simulink model "vel_pose_connect_sl"  (R2018b)
settings: Solver=VariableStepAuto  StartTime=0.0  StopTime=inf  RelTol=1e-3
undefined symbols (not defined in the file or in its folder): Angle, Brakepedal, Drivemode, Drivepedal, Gearshift, Header, Lamp, Light, Speed, Steeringmode, Tm, Twist
libraries: robotlib x19, simulink x3
settings Model: Creator=handai  LastModifiedBy=sdd

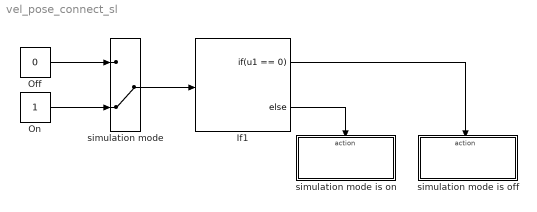
== system vel_pose_connect_sl ==
  If1 : If  IfExpression=u1 == 0
  Off : Constant  Value=0
  On : Constant
  simulation mode : ManualSwitch  CurrentSetting=0
  simulation mode is off : Subsystem  TreatAsAtomicUnit=on
  simulation mode is on : Subsystem  TreatAsAtomicUnit=on
  wires:
  Off/1 -> simulation mode/1
  On/1 -> simulation mode/2
  simulation mode/1 -> If1/1
  If1/1 -> simulation mode is off/Action
  If1/2 -> simulation mode is on/Action

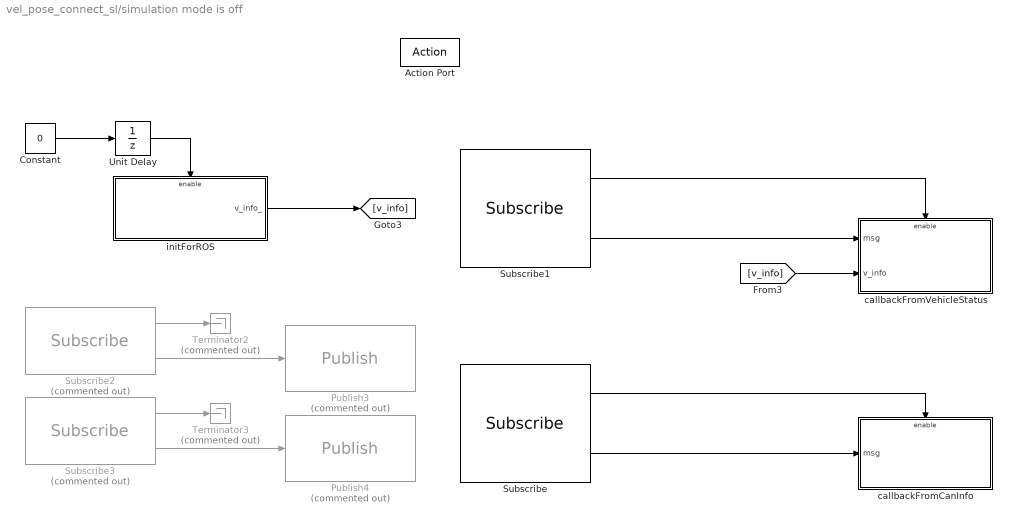
== system vel_pose_connect_sl/simulation mode is off ==
  Action Port : ActionPort  ActionType=then
  Constant : Constant  Value=0
  Publish3 : robotlib/Publish  Commented=on  topicSource=Specify your own  topic=/current_pose  messageType=geometry_msgs/PoseStamped  messageQueueLength=1
      settings: SourceProductBaseCode=RO
  Publish4 : robotlib/Publish  Commented=on  topicSource=Specify your own  topic=/current_velocity  messageType=geometry_msgs/TwistStamped  messageQueueLength=1
      settings: SourceProductBaseCode=RO
  Subscribe : robotlib/Subscribe  topicSource=Specify your own  topic=/can_info  messageType=autoware_msgs/CanInfo  sampleTime=-1  messageQueueLength=1
      settings: SourceProductBaseCode=RO
  Subscribe1 : robotlib/Subscribe  topicSource=Specify your own  topic=/vehicle_status  messageType=autoware_msgs/VehicleStatus  sampleTime=-1  messageQueueLength=1
      settings: SourceProductBaseCode=RO
  Subscribe2 : robotlib/Subscribe  Commented=on  topicSource=Specify your own  topic=/ndt_pose  messageType=geometry_msgs/PoseStamped  sampleTime=-1  messageQueueLength=1
      settings: SourceProductBaseCode=RO
  Subscribe3 : robotlib/Subscribe  Commented=on  topicSource=Specify your own  topic=/estimate_twist  messageType=geometry_msgs/TwistStamped  sampleTime=-1  messageQueueLength=1
      settings: SourceProductBaseCode=RO
  Terminator2 : Terminator  Commented=on
  Terminator3 : Terminator  Commented=on
  Unit Delay : UnitDelay  InitialCondition=1  SampleTime=-1
  callbackFromCanInfo : Subsystem
  callbackFromVehicleStatus : Subsystem
  initForROS : Subsystem
  wires:
  Subscribe2/2 -> Publish3/1
  Subscribe3/2 -> Publish4/1
  Subscribe2/1 -> Terminator2/1
  Subscribe3/1 -> Terminator3/1
  Subscribe/2 -> callbackFromCanInfo/1(msg)
  Subscribe/1 -> callbackFromCanInfo/Enable
  Subscribe1/2 -> callbackFromVehicleStatus/1(msg)
  Subscribe1/1 -> callbackFromVehicleStatus/Enable
  [v_info] -> callbackFromVehicleStatus/2(v_info)
  Constant/1 -> Unit Delay/1
  initForROS/1(v_info_) -> [v_info]
  Unit Delay/1 -> initForROS/Enable

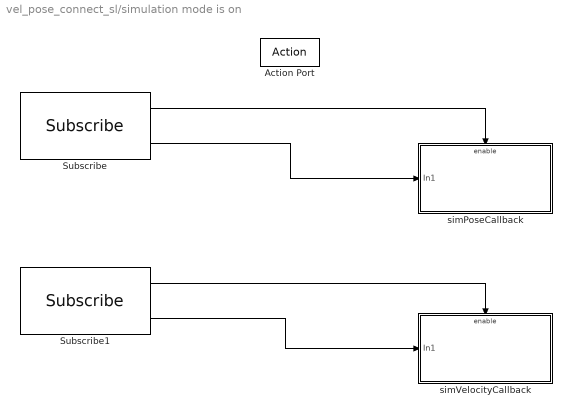
== system vel_pose_connect_sl/simulation mode is on ==
  Action Port : ActionPort  ActionType=else
  Subscribe : robotlib/Subscribe  topicSource=Specify your own  topic=/sim_pose  messageType=geometry_msgs/PoseStamped  sampleTime=-1  messageQueueLength=1
      settings: SourceProductBaseCode=RO
  Subscribe1 : robotlib/Subscribe  topicSource=Specify your own  topic=/sim_velocity  messageType=geometry_msgs/TwistStamped  sampleTime=-1  messageQueueLength=1
      settings: SourceProductBaseCode=RO
  simPoseCallback : Subsystem
  simVelocityCallback : Subsystem
  wires:
  Subscribe/1 -> simPoseCallback/Enable
  Subscribe1/1 -> simVelocityCallback/Enable
  Subscribe/2 -> simPoseCallback/1(In1)
  Subscribe1/2 -> simVelocityCallback/1(In1)

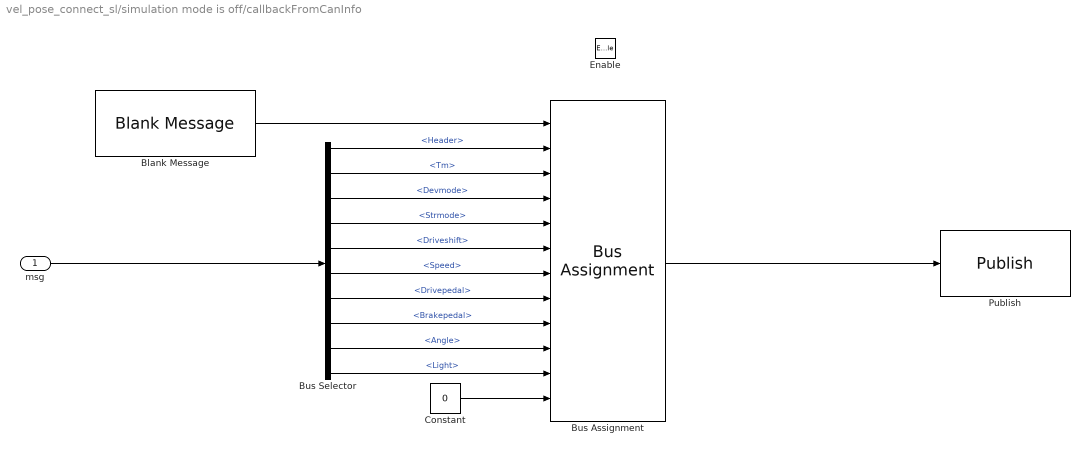
== system vel_pose_connect_sl/simulation mode is off/callbackFromCanInfo ==
  msg : Inport
  Enable : EnablePort
  Blank Message : robotlib/Blank Message  messageClass=Message  entityType=autoware_msgs/VehicleStatus  messageType=autoware_msgs/VehicleStatus  SampleTime=inf
      settings: SourceProductBaseCode=RO
  Bus Assignment : BusAssignment  AssignedSignals=Header,Tm,Drivemode,Steeringmode,Gearshift,Speed,Drivepedal,Brakepedal,Angle,Light,Lamp
  Bus Selector : BusSelector  OutputSignals=Header,Tm,Devmode,Strmode,Driveshift,Speed,Drivepedal,Brakepedal,Angle,Light
  Constant : Constant  Value=0  OutDataTypeStr=int32
  Publish : robotlib/Publish  topicSource=Specify your own  topic=/vehicle_status  messageType=autoware_msgs/VehicleStatus  messageQueueLength=1
      settings: SourceProductBaseCode=RO
  wires:
  Bus Selector/10 -> Bus Assignment/11  "<Light>"
  Bus Assignment/1 -> Publish/1
  Bus Selector/3 -> Bus Assignment/4  "<Devmode>"
  Bus Selector/5 -> Bus Assignment/6  "<Driveshift>"
  msg/1 -> Bus Selector/1
  Bus Selector/2 -> Bus Assignment/3  "<Tm>"
  Bus Selector/1 -> Bus Assignment/2  "<Header>"
  Constant/1 -> Bus Assignment/12
  Bus Selector/9 -> Bus Assignment/10  "<Angle>"
  Bus Selector/6 -> Bus Assignment/7  "<Speed>"
  Bus Selector/7 -> Bus Assignment/8  "<Drivepedal>"
  Bus Selector/8 -> Bus Assignment/9  "<Brakepedal>"
  Bus Selector/4 -> Bus Assignment/5  "<Strmode>"
  Blank Message/1 -> Bus Assignment/1

== system vel_pose_connect_sl/simulation mode is off/callbackFromVehicleStatus ==
  msg : Inport
  v_info : Inport  Port=2
  Enable : EnablePort
  publishVelocity : Subsystem  TreatAsAtomicUnit=on
  publishVelocityViz : Subsystem  TreatAsAtomicUnit=on
  wires:
  msg/1 -> publishVelocity/1(msg), publishVelocityViz/1(msg)
  v_info/1 -> publishVelocity/2(v_info)

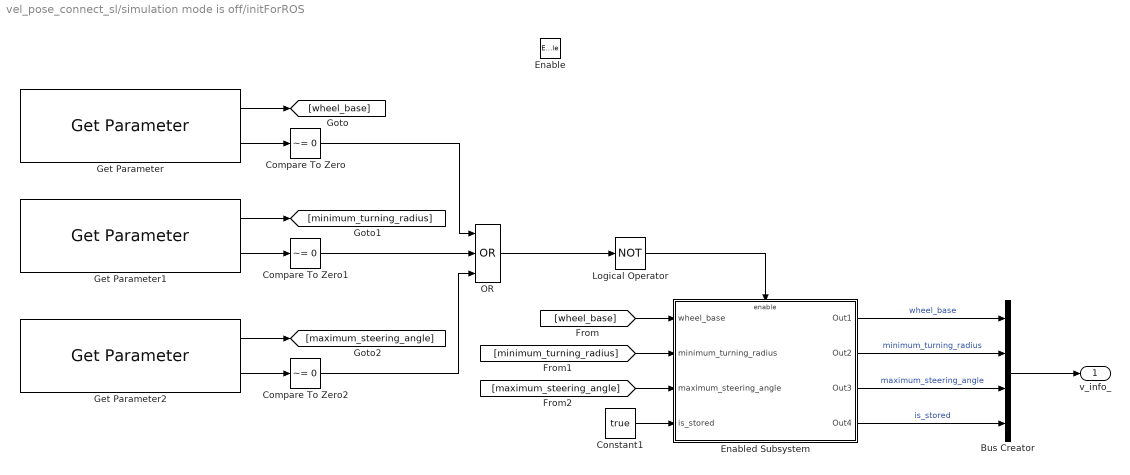
== system vel_pose_connect_sl/simulation mode is off/initForROS ==
  Enable : EnablePort
  Bus Creator : BusCreator  Inputs=4
  Compare To Zero : simulink/Logic and Bit Operations/Compare To Zero  relop=~=  OutDataTypeStr=boolean
  Compare To Zero1 : simulink/Logic and Bit Operations/Compare To Zero  relop=~=  OutDataTypeStr=boolean
  Compare To Zero2 : simulink/Logic and Bit Operations/Compare To Zero  relop=~=  OutDataTypeStr=boolean
  Constant1 : Constant  Value=true  OutDataTypeStr=boolean
  Enabled Subsystem : Subsystem  TreatAsAtomicUnit=on
  Get Parameter : robotlib/Get Parameter  ParameterSource=Specify your own  ParameterName=/vehicle_info/wheel_base  ParameterType=double  ParameterMaxArrayLength=16  ParameterInitialValue=0.0  SampleTime=-1  ShowErrorCodeOutput=on  ModelName=vel_pose_connect_sl  BlockId=ParamGet_vel_pose_connect_sl_17
      settings: SourceProductName=Robotics System Toolbox  SourceProductBaseCode=RO
  Get Parameter1 : robotlib/Get Parameter  ParameterSource=Specify your own  ParameterName=/vehicle_info/minimum_turning_radius  ParameterType=double  ParameterMaxArrayLength=16  ParameterInitialValue=0.0  SampleTime=-1  ShowErrorCodeOutput=on  ModelName=vel_pose_connect_sl  BlockId=ParamGet_vel_pose_connect_sl_18
      settings: SourceProductName=Robotics System Toolbox  SourceProductBaseCode=RO
  Get Parameter2 : robotlib/Get Parameter  ParameterSource=Specify your own  ParameterName=/vehicle_info/maximum_steering_angle  ParameterType=double  ParameterMaxArrayLength=16  ParameterInitialValue=0.0  SampleTime=-1  ShowErrorCodeOutput=on  ModelName=vel_pose_connect_sl  BlockId=ParamGet_vel_pose_connect_sl_19
      settings: SourceProductName=Robotics System Toolbox  SourceProductBaseCode=RO
  Logical Operator : Logic  Operator=NOT  AllPortsSameDT=off  OutDataTypeStr=boolean
  OR : Logic  Operator=OR  Inputs=3  AllPortsSameDT=off  OutDataTypeStr=boolean
  v_info_ : Outport
  wires:
  Get Parameter2/1 -> [maximum_steering_angle]
  Get Parameter1/2 -> Compare To Zero1/1
  OR/1 -> Logical Operator/1
  [wheel_base] -> Enabled Subsystem/1(wheel_base)
  Enabled Subsystem/1(Out1) -> Bus Creator/1  "wheel_base"
  Compare To Zero/1 -> OR/1
  [minimum_turning_radius] -> Enabled Subsystem/2(minimum_turning_radius)
  Constant1/1 -> Enabled Subsystem/4(is_stored)
  Enabled Subsystem/2(Out2) -> Bus Creator/2  "minimum_turning_radius"
  Compare To Zero1/1 -> OR/2
  Enabled Subsystem/3(Out3) -> Bus Creator/3  "maximum_steering_angle"
  [maximum_steering_angle] -> Enabled Subsystem/3(maximum_steering_angle)
  Get Parameter1/1 -> [minimum_turning_radius]
  Get Parameter2/2 -> Compare To Zero2/1
  Enabled Subsystem/4(Out4) -> Bus Creator/4  "is_stored"
  Logical Operator/1 -> Enabled Subsystem/Enable
  Compare To Zero2/1 -> OR/3
  Get Parameter/1 -> [wheel_base]
  Get Parameter/2 -> Compare To Zero/1
  Bus Creator/1 -> v_info_/1

== system vel_pose_connect_sl/simulation mode is on/simPoseCallback ==
  In1 : Inport
  Enable : EnablePort
  Publish : robotlib/Publish  topicSource=Specify your own  topic=/current_pose  messageType=geometry_msgs/PoseStamped  messageQueueLength=1
      settings: SourceProductBaseCode=RO
  wires:
  In1/1 -> Publish/1

== system vel_pose_connect_sl/simulation mode is on/simVelocityCallback ==
  In1 : Inport
  Enable : EnablePort
  Publish1 : robotlib/Publish  topicSource=Specify your own  topic=/current_velocity  messageType=geometry_msgs/TwistStamped  messageQueueLength=1
      settings: SourceProductBaseCode=RO
  wires:
  In1/1 -> Publish1/1

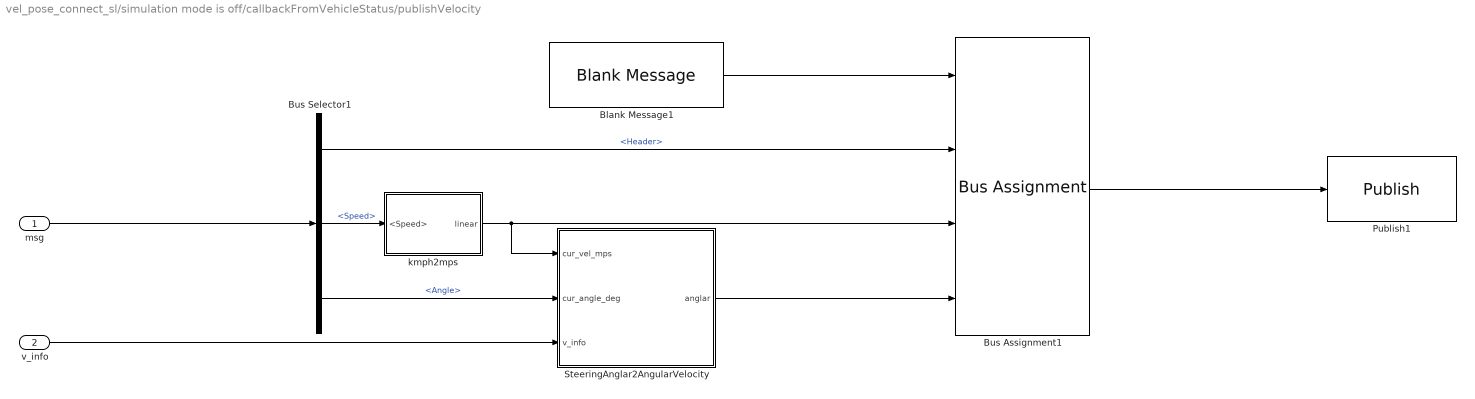
== system vel_pose_connect_sl/simulation mode is off/callbackFromVehicleStatus/publishVelocity ==
  msg : Inport
  v_info : Inport  Port=2
  Blank Message1 : robotlib/Blank Message  messageClass=Message  entityType=geometry_msgs/TwistStamped  messageType=geometry_msgs/TwistStamped  SampleTime=inf
      settings: SourceProductBaseCode=RO
  Bus Assignment1 : BusAssignment  AssignedSignals=Header,Twist.Linear.X,Twist.Angular.Z
  Bus Selector1 : BusSelector  OutputSignals=Header,Speed,Angle
  Publish1 : robotlib/Publish  topicSource=Specify your own  topic=/can_velocity  messageType=geometry_msgs/TwistStamped  messageQueueLength=1
      settings: SourceProductBaseCode=RO
  SteeringAnglar2AngularVelocity : Subsystem  TreatAsAtomicUnit=on
  kmph2mps : Subsystem  TreatAsAtomicUnit=on
  wires:
  Blank Message1/1 -> Bus Assignment1/1
  Bus Assignment1/1 -> Publish1/1
  kmph2mps/1(linear) -> SteeringAnglar2AngularVelocity/1(cur_vel_mps), Bus Assignment1/3
  Bus Selector1/1 -> Bus Assignment1/2  "<Header>"
  Bus Selector1/2 -> kmph2mps/1(<Speed>)  "<Speed>"
  msg/1 -> Bus Selector1/1
  Bus Selector1/3 -> SteeringAnglar2AngularVelocity/2(cur_angle_deg)  "<Angle>"
  v_info/1 -> SteeringAnglar2AngularVelocity/3(v_info)
  SteeringAnglar2AngularVelocity/1(anglar) -> Bus Assignment1/4

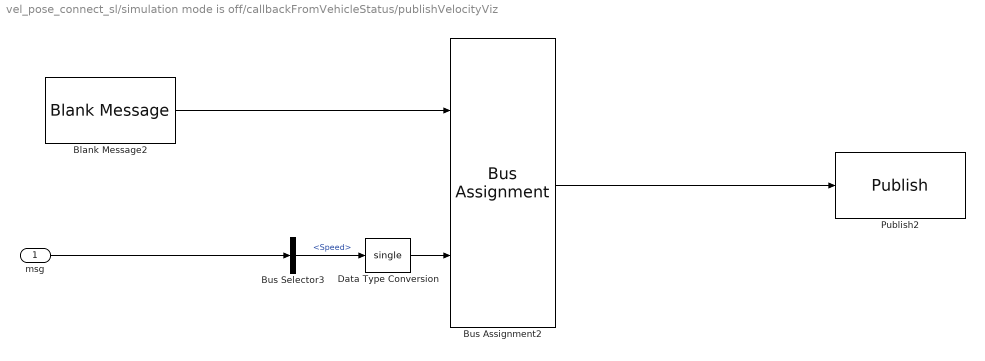
== system vel_pose_connect_sl/simulation mode is off/callbackFromVehicleStatus/publishVelocityViz ==
  msg : Inport
  Blank Message2 : robotlib/Blank Message  messageClass=Message  entityType=std_msgs/Float32  messageType=std_msgs/Float32  SampleTime=inf
      settings: SourceProductBaseCode=RO
  Bus Assignment2 : BusAssignment  AssignedSignals=Data
  Bus Selector3 : BusSelector  OutputSignals=Speed
  Data Type Conversion : DataTypeConversion  OutDataTypeStr=single
  Publish2 : robotlib/Publish  topicSource=Specify your own  topic=/linear_velocity_viz  messageType=std_msgs/Float32  messageQueueLength=1
      settings: SourceProductBaseCode=RO
  wires:
  Bus Assignment2/1 -> Publish2/1
  Data Type Conversion/1 -> Bus Assignment2/2
  Bus Selector3/1 -> Data Type Conversion/1  "<Speed>"
  Blank Message2/1 -> Bus Assignment2/1
  msg/1 -> Bus Selector3/1

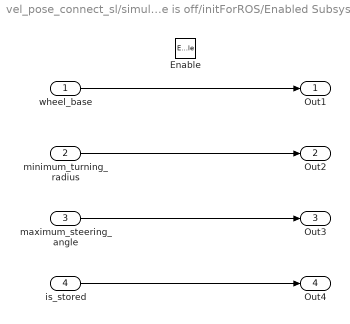
== system vel_pose_connect_sl/simulation mode is off/initForROS/Enabled Subsystem ==
  wheel_base : Inport
  minimum_turning_radius : Inport  Port=2
  maximum_steering_angle : Inport  Port=3
  is_stored : Inport  Port=4
  Enable : EnablePort
  Out1 : Outport  InitialOutput=0
      settings: AttributesFormatString=initial_value = %<InitialOutput>
  Out2 : Outport  Port=2  InitialOutput=0
      settings: AttributesFormatString=initial_value = %<InitialOutput>
  Out3 : Outport  Port=3  InitialOutput=0
      settings: AttributesFormatString=initial_value = %<InitialOutput>
  Out4 : Outport  Port=4  InitialOutput=false
      settings: AttributesFormatString=initial_value = %<InitialOutput>
  wires:
  wheel_base/1 -> Out1/1
  minimum_turning_radius/1 -> Out2/1
  maximum_steering_angle/1 -> Out3/1
  is_stored/1 -> Out4/1

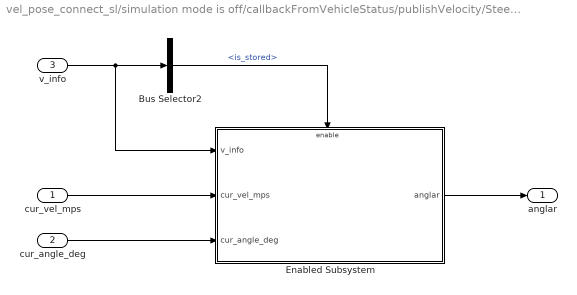
== system vel_pose_connect_sl/simulation mode is off/callbackFromVehicleStatus/publishVelocity/SteeringAnglar2AngularVelocity ==
  cur_vel_mps : Inport
  cur_angle_deg : Inport  Port=2
  v_info : Inport  Port=3
  Bus Selector2 : BusSelector  OutputSignals=is_stored
  Enabled Subsystem : Subsystem  TreatAsAtomicUnit=on
  anglar : Outport
  wires:
  Bus Selector2/1 -> Enabled Subsystem/Enable  "<is_stored>"
  v_info/1 -> Enabled Subsystem/1(v_info), Bus Selector2/1
  Enabled Subsystem/1(anglar) -> anglar/1
  cur_angle_deg/1 -> Enabled Subsystem/3(cur_angle_deg)
  cur_vel_mps/1 -> Enabled Subsystem/2(cur_vel_mps)

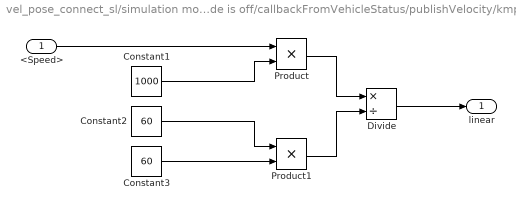
== system vel_pose_connect_sl/simulation mode is off/callbackFromVehicleStatus/publishVelocity/kmph2mps ==
  <Speed> : Inport
  Constant1 : Constant  Value=1000
  Constant2 : Constant  Value=60
  Constant3 : Constant  Value=60
  Divide : Product  Inputs=*/
  Product : Product
  Product1 : Product
  linear : Outport
  wires:
  Constant1/1 -> Product/2
  Constant2/1 -> Product1/1
  Constant3/1 -> Product1/2
  <Speed>/1 -> Product/1
  Divide/1 -> linear/1
  Product/1 -> Divide/1
  Product1/1 -> Divide/2

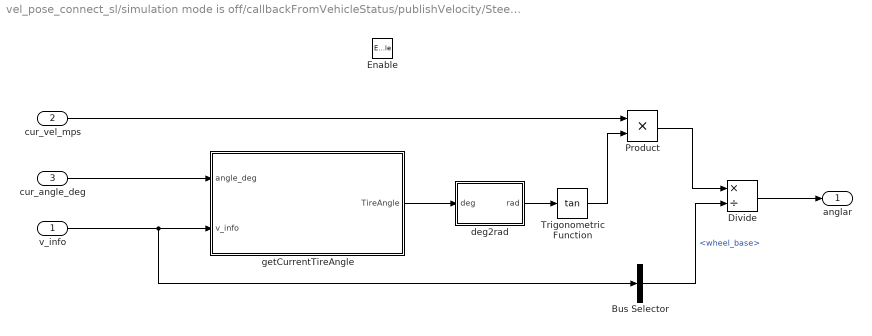
== system vel_pose_connect_sl/simulation mode is off/callbackFromVehicleStatus/publishVelocity/SteeringAnglar2AngularVelocity/Enabled Subsystem ==
  v_info : Inport
  cur_vel_mps : Inport  Port=2
  cur_angle_deg : Inport  Port=3
  Enable : EnablePort  StatesWhenEnabling=reset
  Bus Selector : BusSelector  OutputSignals=wheel_base
  Divide : Product  Inputs=*/
  Product : Product
  Trigonometric Function : Trigonometry  Operator=tan
  deg2rad : Subsystem
  getCurrentTireAngle : Subsystem
  anglar : Outport  OutputWhenDisabled=reset  InitialOutput=0
      settings: AttributesFormatString=|
      | init_value = %<InitialOutput>
      | OutputWhenDisabled = %<OutputWhenDisabled>
  wires:
  deg2rad/1(rad) -> Trigonometric Function/1
  Trigonometric Function/1 -> Product/2
  Product/1 -> Divide/1
  cur_vel_mps/1 -> Product/1
  Divide/1 -> anglar/1
  getCurrentTireAngle/1(TireAngle) -> deg2rad/1(deg)
  v_info/1 -> Bus Selector/1, getCurrentTireAngle/2(v_info)
  cur_angle_deg/1 -> getCurrentTireAngle/1(angle_deg)
  Bus Selector/1 -> Divide/2  "<wheel_base>"

== system vel_pose_connect_sl/simulation mode is off/callbackFromVehicleStatus/publishVelocity/SteeringAnglar2AngularVelocity/Enabled Subsystem/deg2rad ==
  deg : Inport
  Constant : Constant  Value=180
  Divide : Product  Inputs=*/
  Gain : Gain  Gain=pi
  rad : Outport
  wires:
  Constant/1 -> Divide/2
  deg/1 -> Gain/1
  Gain/1 -> Divide/1
  Divide/1 -> rad/1

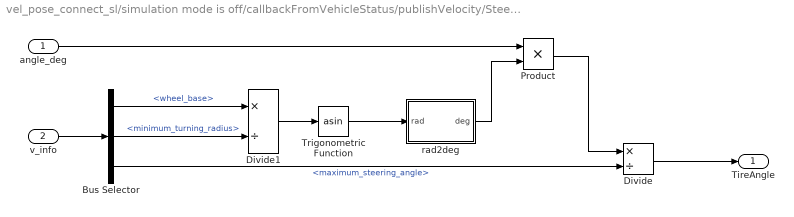
== system vel_pose_connect_sl/simulation mode is off/callbackFromVehicleStatus/publishVelocity/SteeringAnglar2AngularVelocity/Enabled Subsystem/getCurrentTireAngle ==
  angle_deg : Inport
  v_info : Inport  Port=2
  Bus Selector : BusSelector  OutputSignals=wheel_base,minimum_turning_radius,maximum_steering_angle
  Divide : Product  Inputs=*/
  Divide1 : Product  Inputs=*/
  Product : Product
  Trigonometric Function : Trigonometry  Operator=asin
  rad2deg : Subsystem
  TireAngle : Outport
  wires:
  Product/1 -> Divide/1
  rad2deg/1(deg) -> Product/2
  Divide/1 -> TireAngle/1
  angle_deg/1 -> Product/1
  Divide1/1 -> Trigonometric Function/1
  Trigonometric Function/1 -> rad2deg/1(rad)
  v_info/1 -> Bus Selector/1
  Bus Selector/2 -> Divide1/2  "<minimum_turning_radius>"
  Bus Selector/1 -> Divide1/1  "<wheel_base>"
  Bus Selector/3 -> Divide/2  "<maximum_steering_angle>"

== system vel_pose_connect_sl/simulation mode is off/callbackFromVehicleStatus/publishVelocity/SteeringAnglar2AngularVelocity/Enabled Subsystem/getCurrentTireAngle/rad2deg ==
  rad : Inport
  Divide1 : Product  Inputs=*/
  Gain : Gain  Gain=180
  Pi : Constant  Value=pi  OutDataTypeStr=Inherit: Inherit via back propagation
  deg : Outport
  wires:
  Pi/1 -> Divide1/2
  Gain/1 -> Divide1/1
  rad/1 -> Gain/1
  Divide1/1 -> deg/1
